simulink model "RotaryWingSim"  (Simulink 4.00)
settings: Solver=ode15s  StartTime=0.0  StopTime=simTime  RelTol=1e-10
values from neighbouring files (symbols this model uses):
  A1STrim = A1S    [AcFrcMmtSummationOutF.m]    (also in RotaryWingSimStart.m = AB1CP(1) + A1CL)
  B1STrim = B1S    [AcFrcMmtSummationOutF.m]    (also in RotaryWingSimStart.m = AB1CP(2) + B1CL)
  C5 = dthetomddelc    [RotaryWingSimStart.m]
  dla = u(2)    [D2ABcpSfunc.m]    (also in RotaryWingSimStart.m = trmOut(3))
  dlc = trmOut(1)    [RotaryWingSimStart.m]
  dlcTrim = dlc    [RotaryWingSimStart.m]
  dle = u(1)    [D2ABcpSfunc.m]    (also in HorizStabFrcMmtSFunc.m = u(7); RotaryWingSimStart.m = trmOut(2))
  dlp = u(7)    [FinFrcMmtSFunc.m]    (also in RotaryWingSimStart.m = trmOut(4); TailRotorFrcMmtSFunc.m)
  dlt = u(4)    [PropellerFrcMmtSFunc.m]    (also in RotaryWingSimStart.m = trmOut(5); acTrim3DFM.m = real(deltt(i)))
  fZMRTrim = -trmOut(9)    [RotaryWingSimStart.m]
  gamRot = 10    [LongitudinalStabilityBensen.m]    (also in N6NNeval.m = 12.5; RotaryWingSimStart.m = gamRot*rhoAir/rhoAirN)
  kB = K_l*tauB    [RotaryWingSimStart.m]
  oMTrim = trmOut(8)    [RotaryWingSimStart.m]
  phiTrim = trmOut(6)    [RotaryWingSimStart.m]
  psiTrim = aE(3)    [RotaryWingSimStart.m]
  tauAgLp = 1.0e-12    (= 1e-12)    [RotaryWingSimStart.m]
  thtaTrim = trmOut(7)    [RotaryWingSimStart.m]
  vE = [xh,0,0]    [RotaryWingSimStart.m]    (also in ac6DofFunc.m = vOut(2))
undefined symbols (not defined in the file or in its folder): A1CL, B1CL, d2ABCP, dlaStp, dlcStp, dleStp, dlpStp, dTstp, fStp1, PIDcllt, PIDphi, PIDpsi, PIDthta, tauB, tauC, tStp, uBStrt, vBStrt, wBStrt
libraries: simulink3 x1
settings Model: LastModifiedBy=jhumt  SaveState=on  InitialState=xFinal  SaveFinalState=on  RTWOptions="-aEnforceIntegerDowncast=1 -aExtMode=0 -aFoldNonRolledExpr=1 -aForceParamTrailComments=0 -aGenerateComments=1 -aIgnoreCustomStorageClasses=1 -aIncHierarchyInIds=0 -aInlineInvariantSignals=0 -aLocalBlockOutputs=1 -aLogVarNameModifier=\"rt_\" -aRTWVerbose=1 -aRollThreshold=5 -aShowEliminatedStatements=1"

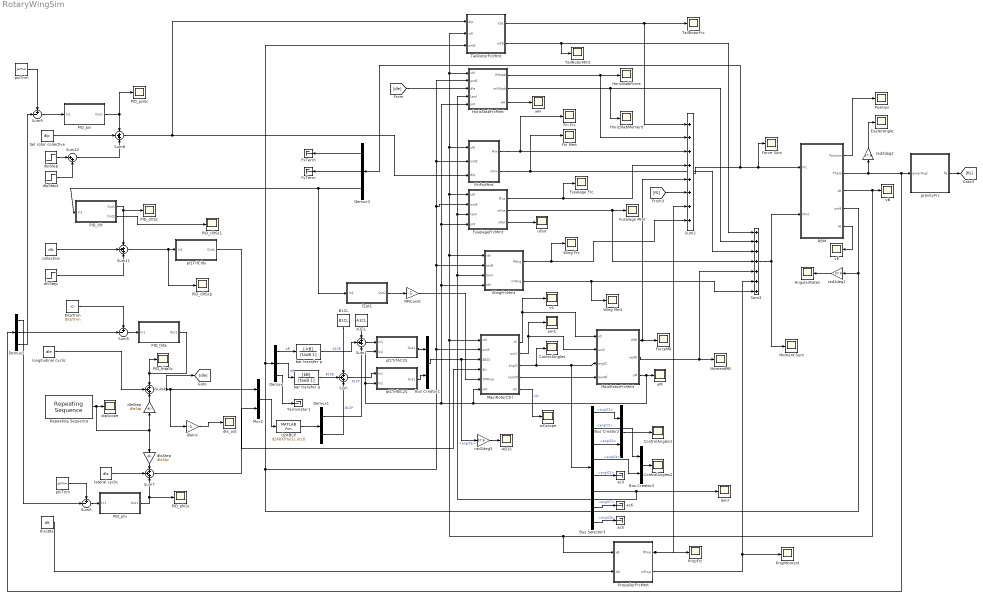
== system RotaryWingSim ==
  A1CL : Constant  Orientation=down  Value=A1CL
  AB1S : Scope
      settings: TimeRange=auto  YMin=-13  YMax=0  SaveToWorkspace=off  SaveName=ScopeData4  LimitDataPoints=on  MaxDataPoints=5000
  AngularRates : Scope
      settings: TimeRange=20  YMin=-12.5  YMax=15  SaveToWorkspace=off  SaveName=ScopeData20  LimitDataPoints=on  MaxDataPoints=25000
  B1CL : Constant  Orientation=down  Value=B1CL
  Bus Creator1 : BusCreator  Inputs=2
  Bus Creator2 : BusCreator  Inputs=2
  Bus Creator3 : BusCreator  Inputs=2
  Bus Selector3 : BusSelector  OutputSignals=anglC1,anglC2,anglC3,anglC4,anglC5,anglC6,anglC7,anglC8  MuxedOutput=off
  ControlAngles : Scope
      settings: TimeRange=auto  YMin=-0.035  YMax=0.065  SaveToWorkspace=off  LimitDataPoints=on  MaxDataPoints=5000
  ControlAngles1 : Scope
      settings: TimeRange=auto  YMin=0.043  YMax=0.064  SaveToWorkspace=off  SaveName=ScopeData33  LimitDataPoints=on  MaxDataPoints=5000
  ControlAngles2 : Scope
      settings: TimeRange=auto  YMin=-0.07  YMax=0.13  SaveToWorkspace=off  SaveName=ScopeData34  LimitDataPoints=on  MaxDataPoints=5000
  Demux : Demux  Outputs=3  BusSelectionMode=off
  Demux1 : Demux  Outputs=2  BusSelectionMode=off
  Demux2 : Demux  Outputs=3  BusSelectionMode=off
  Demux3 : Demux  Orientation=left  Outputs=3  BusSelectionMode=off
  EuelerAngle : Scope
      settings: TimeRange=auto  YMin=-7  YMax=7  SaveToWorkspace=off  SaveName=ScopeData17  LimitDataPoints=on  MaxDataPoints=25000
  Fin Frc : Scope
      settings: TimeRange=auto  YMin=-200  YMax=150  SaveToWorkspace=off  SaveName=ScopeData12  LimitDataPoints=on  MaxDataPoints=5000
  Fin Mmt : Scope
      settings: TimeRange=auto  YMin=-5  YMax=5  SaveToWorkspace=off  SaveName=ScopeData13  LimitDataPoints=on  MaxDataPoints=25000
  FinFrcMmt : Subsystem
      settings: RTWFcnNameOpts=Auto  RTWFileNameOpts=Auto
  Force Sum : Scope
      settings: TimeRange=0.02560000000000007  YMin=-0.0507109  YMax=0.0687204  SaveToWorkspace=off  SaveName=ScopeData15  LimitDataPoints=on  MaxDataPoints=5000
  ForceMR : Scope
      settings: TimeRange=30  YMin=-80000  YMax=5000  SaveToWorkspace=off  SaveName=ScopeData6  LimitDataPoints=on  MaxDataPoints=5000
  Fuselage Frc : Scope
      settings: TimeRange=auto  YMin=-5  YMax=5  SaveToWorkspace=off  SaveName=ScopeData10  LimitDataPoints=on  MaxDataPoints=5000
  Fuselage Mmt : Scope
      settings: TimeRange=auto  YMin=-175  YMax=25  SaveToWorkspace=off  SaveName=ScopeData11  LimitDataPoints=on  MaxDataPoints=5000
  FuselageFrcMmt : Subsystem
      settings: RTWFcnNameOpts=Auto  RTWFileNameOpts=Auto
  FxTerm : Terminator
  FyTerm : Terminator
  HorizStabForce : Scope
      settings: TimeRange=auto  YMin=-100  YMax=1200  SaveToWorkspace=off  SaveName=ScopeData18  LimitDataPoints=on  MaxDataPoints=5000
  HorizStabFrcMmt : Subsystem
      settings: RTWFcnNameOpts=Auto  RTWFileNameOpts=Auto
  HorizStabMoment : Scope
      settings: TimeRange=auto  YMin=0  YMax=450  SaveToWorkspace=off  SaveName=ScopeData19  LimitDataPoints=on  MaxDataPoints=25000
  MRConst : Gain  Gain=-1  Multiplication=Element-wise(K.*u)  SaturateOnIntegerOverflow=on
  MainRotorCtrl : Subsystem
      settings: RTWFcnNameOpts=Auto  RTWFileNameOpts=Auto
  MainRotorFrcMmt : Subsystem
      settings: RTWFcnNameOpts=Auto  RTWFileNameOpts=Auto
  Moment Sum : Scope
      settings: TimeRange=auto  YMin=-5  YMax=45  SaveToWorkspace=off  SaveName=ScopeData14  LimitDataPoints=on  MaxDataPoints=5000
  MomentMR : Scope
      settings: TimeRange=auto  YMin=-2250  YMax=500  SaveToWorkspace=off  SaveName=ScopeData5  LimitDataPoints=on  MaxDataPoints=25000
  Mux2 : Mux  Inputs=2
  PID_cllt : Subsystem
      settings: RTWFcnNameOpts=Auto  RTWFileNameOpts=Auto
  PID_clltSc : Scope
      settings: TimeRange=auto  YMin=-1  YMax=1  SaveToWorkspace=off  SaveName=ScopeData29  LimitDataPoints=on  MaxDataPoints=5000
  PID_clltSc1 : Scope
      settings: TimeRange=auto  YMin=-26  YMax=-15  SaveToWorkspace=off  SaveName=ScopeData30  LimitDataPoints=on  MaxDataPoints=5000
  PID_clltScp : Scope
      settings: TimeRange=auto  YMin=0.19401  YMax=0.19407  SaveToWorkspace=off  SaveName=ScopeData22  LimitDataPoints=on  MaxDataPoints=5000
  PID_phi : Subsystem
      settings: RTWFcnNameOpts=Auto  RTWFileNameOpts=Auto
  PID_phiSc : Scope
      settings: TimeRange=auto  YMin=-5  YMax=5  SaveToWorkspace=off  SaveName=ScopeData26  LimitDataPoints=on  MaxDataPoints=5000
  PID_psi : Subsystem
      settings: RTWFcnNameOpts=Auto  RTWFileNameOpts=Auto
  PID_psiSc : Scope
      settings: TimeRange=auto  YMin=-0.015  YMax=0.0025  SaveToWorkspace=off  SaveName=ScopeData25  LimitDataPoints=on  MaxDataPoints=5000
  PID_thta : Subsystem
      settings: RTWFcnNameOpts=Auto  RTWFileNameOpts=Auto
  PID_thtaSc : Scope
      settings: TimeRange=auto  YMin=-4.5  YMax=1  SaveToWorkspace=off  SaveName=ScopeData24  LimitDataPoints=on  MaxDataPoints=5000
  Position : Scope
      settings: TimeRange=auto  YMin=-500  YMax=1500  SaveToWorkspace=off  SaveName=ScopeData16  LimitDataPoints=on  MaxDataPoints=25000
  PropFrc : Scope
      settings: TimeRange=auto  YMin=0  YMax=350  SaveToWorkspace=off  SaveName=ScopeData36  LimitDataPoints=on  MaxDataPoints=5000
  PropMoment : Scope
      settings: TimeRange=auto  YMin=0  YMax=15  SaveToWorkspace=off  SaveName=ScopeData35  LimitDataPoints=on  MaxDataPoints=5000
  PropellerFrcMmt : Subsystem
      settings: RTWFcnNameOpts=Auto  RTWFileNameOpts=Auto
  RBM : Subsystem
      settings: RTWFcnNameOpts=Auto  RTWFileNameOpts=Auto
  Repeating Sequence : simulink3/Sources/Repeating Sequence  rep_seq_t=fStp1(1,:)  rep_seq_y=fStp1(2,:)
  Sum{,1,4,7..8,11} (6 alike) : Sum  Inputs=+++  SaturateOnIntegerOverflow=on
  Sum12 : Sum  Inputs=|++  SaturateOnIntegerOverflow=on
  Sum2 : Sum  Inputs=++++++++  SaturateOnIntegerOverflow=on
  Sum3 : Sum  Inputs=+++++++  SaturateOnIntegerOverflow=on
  Sum5 : Sum  Inputs=+-|  SaturateOnIntegerOverflow=on
  Sum6 : Sum  Inputs=+-|  SaturateOnIntegerOverflow=on
  Sum9 : Sum  Inputs=+-|  SaturateOnIntegerOverflow=on
  TailRotorFrc : Scope
      settings: TimeRange=auto  YMin=-5  YMax=5  SaveToWorkspace=off  SaveName=ScopeData8  LimitDataPoints=on  MaxDataPoints=5000
  TailRotorFrcMmt : Subsystem
      settings: RTWFcnNameOpts=Auto  RTWFileNameOpts=Auto
  TailRotorMmt : Scope
      settings: TimeRange=auto  YMin=-50000  YMax=200000  SaveToWorkspace=off  SaveName=ScopeData9  LimitDataPoints=on  MaxDataPoints=5000
  Terminator1 : Terminator
  Wing Frc : Scope
      settings: TimeRange=auto  YMin=-1750  YMax=0  SaveToWorkspace=off  SaveName=ScopeData39  LimitDataPoints=on  MaxDataPoints=5000
  Wing Mmt : Scope
      settings: TimeRange=auto  YMin=-7.5  YMax=15  SaveToWorkspace=off  SaveName=ScopeData38  LimitDataPoints=on  MaxDataPoints=5000
  WingFrcMmt : Subsystem
      settings: RTWFcnNameOpts=Auto  RTWFileNameOpts=Auto
  ac3 : Terminator
  ac5 : Terminator
  ac6 : Terminator
  bar transfer p : TransferFcn  Numerator=[-kB]  Denominator=[tauB 1]  AbsoluteTolerance=auto  Realization=auto
  bar transfer q : TransferFcn  Numerator=[kB]  Denominator=[tauB 1]  AbsoluteTolerance=auto  Realization=auto
  collective : Constant  Value=dlc
  d2ABCP : MATLABFcn  MATLABFcn=d2ABCP(u(1),u(2))  OutputDimensions=-1  OutputSignalType=auto  Output1D=on
  dlaStep : Gain  Orientation=down  Gain=dlaStp  Multiplication=Element-wise(K.*u)  SaturateOnIntegerOverflow=on
  dlcStep : Step  Time=tStp  Before=0  After=dlcStp  SampleTime=0
  dleInv : Gain  Gain=-1  Multiplication=Element-wise(K.*u)  SaturateOnIntegerOverflow=on
  dleStep : Gain  Orientation=up  Gain=dleStp  Multiplication=Element-wise(K.*u)  SaturateOnIntegerOverflow=on
  dle_out : Scope
      settings: TimeRange=auto  YMin=-125  YMax=75  SaveToWorkspace=off  SaveName=ScopeData32  LimitDataPoints=on  MaxDataPoints=15000
  dlpStep : Step  Time=tStp  Before=0  After=dlpStp  SampleTime=0
  dlpStep1 : Step  Time=tStp + dTstp  Before=0  After=- dlpStp  SampleTime=0
  fZpt1 : Subsystem
      settings: RTWFcnNameOpts=Auto  RTWFileNameOpts=Auto
  gravityFrc : Subsystem
      settings: RTWFcnNameOpts=Auto  RTWFileNameOpts=Auto
  lamI : Scope
      settings: TimeRange=auto  YMin=0  YMax=350  SaveToWorkspace=off  SaveName=ScopeData3  LimitDataPoints=on  MaxDataPoints=5000
  lateral cyclic : Constant  Value=dla
  longitudinal cyclic : Constant  Value=dle
  oM : Scope
      settings: TimeRange=auto  YMin=31  YMax=42  SaveToWorkspace=off  SaveName=ScopeData7  LimitDataPoints=on  MaxDataPoints=25000
  omC : Scope
      settings: TimeRange=auto  YMin=-5  YMax=5  SaveToWorkspace=off  SaveName=ScopeData2  LimitDataPoints=on  MaxDataPoints=5000
  phiTrim : Constant  Value=phiTrim
  psiTrim : Constant  Value=psiTrim
  pt1TrfAC2S : Subsystem
      settings: RTWFcnNameOpts=Auto  RTWFileNameOpts=Auto
  pt1TrfBC2S : Subsystem
      settings: RTWFcnNameOpts=Auto  RTWFileNameOpts=Auto
  pt1TrfClltv : Subsystem
      settings: RTWFcnNameOpts=Auto  RTWFileNameOpts=Auto
  rad2deg1 : Gain  Orientation=left  Gain=57.6  Multiplication=Element-wise(K.*u)  SaturateOnIntegerOverflow=on
  rad2deg2 : Gain  Orientation=up  Gain=57.6  Multiplication=Element-wise(K.*u)  SaturateOnIntegerOverflow=on
  rad2deg3 : Gain  Gain=57.6  Multiplication=Element-wise(K.*u)  SaturateOnIntegerOverflow=on
  stpScope : Scope
      settings: TimeRange=auto  YMin=-0.5  YMax=1.2  SaveToWorkspace=off  SaveName=ScopeData37  LimitDataPoints=on  MaxDataPoints=5000
  tail rotor collective : Constant  Value=dlp
  throttle : Constant  Value=dlt
  thtaTrim : Constant  Value=thtaTrim
  uOut : Scope
      settings: TimeRange=auto  YMin=-5  YMax=5  SaveToWorkspace=off  SaveName=ScopeData28  LimitDataPoints=on  MaxDataPoints=5000
  vB : Scope
      settings: TimeRange=auto  YMin=0  YMax=30  SaveToWorkspace=off  SaveName=ScopeData27  LimitDataPoints=on  MaxDataPoints=5000
  vC : Scope
      settings: TimeRange=auto  YMin=-5  YMax=5  SaveToWorkspace=off  SaveName=ScopeData  LimitDataPoints=on  MaxDataPoints=5000
  vE : Scope
      settings: TimeRange=auto  YMin=0  YMax=32.5  SaveToWorkspace=off  SaveName=ScopeData31  LimitDataPoints=on  MaxDataPoints=5000
  wCscope : Scope
      settings: TimeRange=auto  YMin=-5  YMax=5  SaveToWorkspace=off  SaveName=ScopeData21  LimitDataPoints=on  MaxDataPoints=5000
  wH : Scope
      settings: TimeRange=auto  YMin=-5  YMax=5  SaveToWorkspace=off  SaveName=ScopeData23  LimitDataPoints=on  MaxDataPoints=5000
  wires:
  Mux2/1 -> d2ABCP/1
  d2ABCP/1 -> Demux1/1
  Demux/1 -> bar transfer p/1  "pB"
  Demux/2 -> bar transfer q/1  "qB"
  bar transfer p/1 -> Sum1/2  "A1CB"
  bar transfer q/1 -> Sum/2  "B1CB"
  B1CL/1 -> Sum/1
  A1CL/1 -> Sum1/1
  Demux1/1 -> Sum1/3  "A1CP"
  Demux1/2 -> Sum/3  "B1CP"
  Sum1/1 -> pt1TrfAC2S/1(In1)
  Sum/1 -> pt1TrfBC2S/1(In1)
  pt1TrfBC2S/1(Out1) -> Bus Creator1/2
  pt1TrfAC2S/1(Out1) -> Bus Creator1/1
  MainRotorCtrl/4(lamNf) -> MainRotorFrcMmt/4(lamNf)
  pt1TrfClltv/1(Out1) -> MainRotorCtrl/4(dlc)
  Bus Creator1/1 -> MainRotorCtrl/3(AB1S), rad2deg3/1
  Demux/3 -> Terminator1/1
  MainRotorCtrl/1(vC) -> vC/1, MainRotorFrcMmt/1(vC)
  MainRotorCtrl/2(omC) -> omC/1, MainRotorFrcMmt/2(omC)
  MainRotorCtrl/3(anglC) -> ControlAngles/1, MainRotorFrcMmt/3(anglC), Bus Selector3/1
  MainRotorFrcMmt/2(mMR) -> Sum3/5, MomentMR/1
  MainRotorFrcMmt/1(fMR) -> ForceMR/1, Sum2/5
  tail rotor collective/1 -> Sum8/2
  TailRotorFrcMmt/2(mTR) -> Sum3/1, TailRotorMmt/1
  TailRotorFrcMmt/1(fTR) -> Sum2/1, TailRotorFrc/1
  FuselageFrcMmt/1(fFus) -> Sum2/4, Fuselage Frc/1
  FuselageFrcMmt/2(mFus) -> Sum3/4, Fuselage Mmt/1
  FinFrcMmt/1(fFin) -> Fin Frc/1, Sum2/3
  FinFrcMmt/2(mFin) -> Fin Mmt/1, Sum3/3
  [dle] -> HorizStabFrcMmt/3(dle)
  Sum2/1 -> Force Sum/1, RBM/1(Frc), Demux3/1
  HorizStabFrcMmt/1(fHStab) -> Sum2/2, HorizStabForce/1
  HorizStabFrcMmt/2(mHStab) -> Sum3/2, HorizStabMoment/1
  Sum3/1 -> Moment Sum/1, RBM/2(Mmt)
  RBM/2(Theta) -> gravityFrc/1(eulerAngl), Demux2/1, rad2deg2/1
  RBM/1(Position) -> Position/1
  [fG] -> Sum2/6
  gravityFrc/1(fG) -> [fG]
  HorizStabFrcMmt/3(wH) -> wH/1
  Sum4/1 -> [dle], Mux2/1, dleInv/1
  thtaTrim/1 -> Sum5/1
  Sum5/1 -> PID_thta/1(In1)
  Demux2/2 -> Sum5/2
  Demux2/1 -> Sum6/2
  Demux2/3 -> Sum9/2
  PID_thta/1(Out1) -> Sum4/1, PID_thtaSc/1
  phiTrim/1 -> Sum6/1
  Sum6/1 -> PID_phi/1(In1)
  Sum7/1 -> Mux2/2
  PID_phi/1(Out1) -> PID_phiSc/1, Sum7/3
  Sum8/1 -> TailRotorFrcMmt/1(dlp), FinFrcMmt/3(dlp)
  PID_psi/1(Out1) -> Sum8/1, PID_psiSc/1
  Sum9/1 -> PID_psi/1(In1)
  psiTrim/1 -> Sum9/1
  RBM/3(vB) -> vB/1, MainRotorCtrl/1(vW), FuselageFrcMmt/1(vW), FinFrcMmt/1(vW), HorizStabFrcMmt/1(vW), TailRotorFrcMmt/2(vW), WingFrcMmt/1(vW), PropellerFrcMmt/1(vB)
  FuselageFrcMmt/3(uOut) -> uOut/1
  collective/1 -> Sum11/2
  Sum11/1 -> pt1TrfClltv/1(In1), PID_clltScp/1
  PID_cllt/1(Out1) -> Sum11/1, PID_clltSc/1
  Demux3/1 -> FxTerm/1
  Demux3/2 -> FyTerm/1
  Demux3/3 -> PID_cllt/1(In1), fZpt1/1(In1)
  PID_cllt/2(Out2) -> PID_clltSc1/1
  RBM/5(vE) -> vE/1
  longitudinal cyclic/1 -> Sum4/2
  MainRotorCtrl/5(wC) -> wCscope/1  "vZc"
  RBM/4(omB) -> MainRotorCtrl/2(omB), FuselageFrcMmt/2(omB), FinFrcMmt/2(omB), HorizStabFrcMmt/2(omB), WingFrcMmt/2(omB), TailRotorFrcMmt/3(omB), Demux/1, rad2deg1/1
  rad2deg1/1 -> AngularRates/1
  dlcStep/1 -> Sum11/3
  dlpStep1/1 -> Sum12/2
  dlpStep/1 -> Sum12/1
  Sum12/1 -> Sum8/3
  lateral cyclic/1 -> Sum7/2
  dleStep/1 -> Sum4/3
  dlaStep/1 -> Sum7/1
  rad2deg2/1 -> EuelerAngle/1
  throttle/1 -> PropellerFrcMmt/2(dlt)
  PropellerFrcMmt/2(mProp) -> Sum3/6, PropMoment/1
  PropellerFrcMmt/1(fProp) -> Sum2/7, PropFrc/1
  MainRotorFrcMmt/3(oM) -> oM/1, pt1TrfAC2S/2(In2), pt1TrfBC2S/2(In2), WingFrcMmt/4(oM), FuselageFrcMmt/4(oM), HorizStabFrcMmt/5(oM), MainRotorCtrl/6(oM)
  Bus Selector3/5 -> ac3/1  "<anglC5>"
  Bus Selector3/7 -> ac6/1  "<anglC7>"
  Bus Selector3/8 -> ac5/1  "<anglC8>"
  Bus Creator2/1 -> ControlAngles1/1
  Bus Selector3/4 -> Bus Creator3/2  "<anglC4>"
  Bus Selector3/2 -> Bus Creator3/1  "<anglC2>"
  Bus Selector3/1 -> Bus Creator2/1  "<anglC1>"
  Bus Selector3/3 -> Bus Creator2/2  "<anglC3>"
  Bus Creator3/1 -> ControlAngles2/1
  rad2deg3/1 -> AB1S/1
  fZpt1/1(Out1) -> MRConst/1
  MRConst/1 -> MainRotorCtrl/5(TMRinp)
  WingFrcMmt/2(mWng) -> Sum3/7, Wing Mmt/1
  WingFrcMmt/1(fWng) -> Sum2/8, Wing Frc/1
  Repeating Sequence/1 -> stpScope/1, dleStep/1, dlaStep/1
  Bus Selector3/6 -> lamI/1, WingFrcMmt/3("lamI "), FuselageFrcMmt/3(lamI), HorizStabFrcMmt/4(lamI)  "<anglC6>"
  dleInv/1 -> dle_out/1

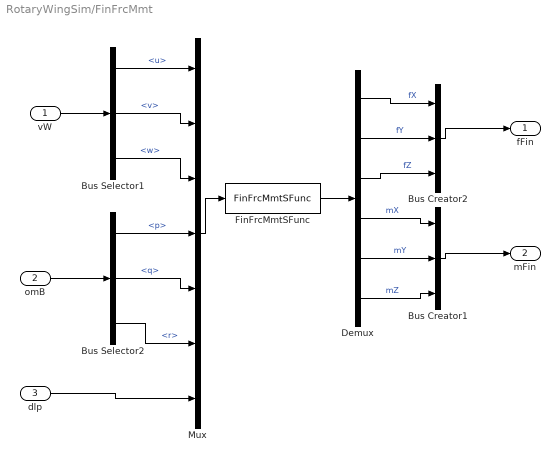
== system RotaryWingSim/FinFrcMmt ==
  vW : Inport  Port=1  LatchInput=off
  omB : Inport  Port=2  LatchInput=off
  dlp : Inport  Port=3  LatchInput=off
  Bus Creator1 : BusCreator  Inputs=3
  Bus Creator2 : BusCreator  Inputs=3
  Bus Selector1 : BusSelector  OutputSignals=u,v,w  MuxedOutput=off
  Bus Selector2 : BusSelector  OutputSignals=p,q,r  MuxedOutput=off
  Demux : Demux  Outputs=6  BusSelectionMode=off
  FinFrcMmtSFunc : S-Function  FunctionName=FinFrcMmtSFunc  PortCounts=[]  SFunctionModules=''
  Mux : Mux  Inputs=7
  fFin : Outport  Port=1
  mFin : Outport  Port=2
  wires:
  vW/1 -> Bus Selector1/1
  Bus Creator2/1 -> fFin/1
  FinFrcMmtSFunc/1 -> Demux/1
  Mux/1 -> FinFrcMmtSFunc/1
  Bus Selector1/2 -> Mux/2  "<v>"
  Bus Selector1/3 -> Mux/3  "<w>"
  omB/1 -> Bus Selector2/1
  Bus Selector2/1 -> Mux/4  "<p>"
  Bus Creator1/1 -> mFin/1
  Demux/1 -> Bus Creator2/1  "fX"
  Demux/2 -> Bus Creator2/2  "fY"
  Demux/3 -> Bus Creator2/3  "fZ"
  Demux/4 -> Bus Creator1/1  "mX"
  Demux/5 -> Bus Creator1/2  "mY"
  Demux/6 -> Bus Creator1/3  "mZ"
  Bus Selector2/2 -> Mux/5  "<q>"
  Bus Selector2/3 -> Mux/6  "<r>"
  Bus Selector1/1 -> Mux/1  "<u>"
  dlp/1 -> Mux/7

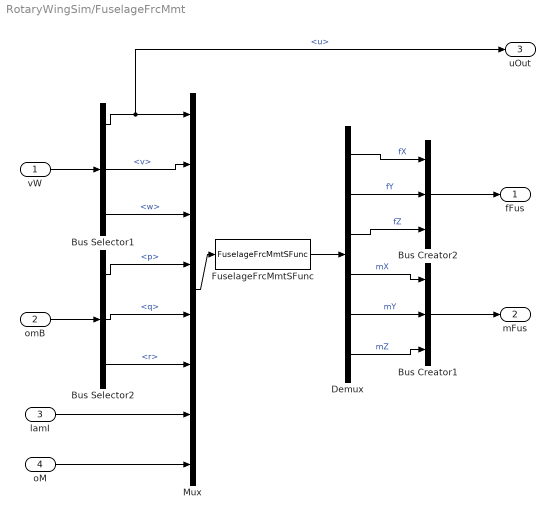
== system RotaryWingSim/FuselageFrcMmt ==
  vW : Inport  Port=1  LatchInput=off
  omB : Inport  Port=2  LatchInput=off
  lamI : Inport  Port=3  LatchInput=off
  oM : Inport  Port=4  LatchInput=off
  Bus Creator1 : BusCreator  Inputs=3
  Bus Creator2 : BusCreator  Inputs=3
  Bus Selector1 : BusSelector  OutputSignals=u,v,w  MuxedOutput=off
  Bus Selector2 : BusSelector  OutputSignals=p,q,r  MuxedOutput=off
  Demux : Demux  Outputs=6  BusSelectionMode=off
  FuselageFrcMmtSFunc : S-Function  FunctionName=FuselageFrcMmtSFunc  PortCounts=[]  SFunctionModules=''
  Mux : Mux  Inputs=8
  fFus : Outport  Port=1
  mFus : Outport  Port=2
  uOut : Outport  Port=3
  wires:
  vW/1 -> Bus Selector1/1
  Bus Creator2/1 -> fFus/1
  FuselageFrcMmtSFunc/1 -> Demux/1
  Mux/1 -> FuselageFrcMmtSFunc/1
  Bus Selector1/1 -> Mux/1, uOut/1  "<u>"
  Bus Selector1/2 -> Mux/2  "<v>"
  omB/1 -> Bus Selector2/1
  Bus Selector2/1 -> Mux/4  "<p>"
  Bus Selector2/2 -> Mux/5  "<q>"
  Bus Selector2/3 -> Mux/6  "<r>"
  Bus Creator1/1 -> mFus/1
  Demux/1 -> Bus Creator2/1  "fX"
  Demux/2 -> Bus Creator2/2  "fY"
  Demux/3 -> Bus Creator2/3  "fZ"
  Demux/4 -> Bus Creator1/1  "mX"
  Demux/5 -> Bus Creator1/2  "mY"
  Demux/6 -> Bus Creator1/3  "mZ"
  Bus Selector1/3 -> Mux/3  "<w>"
  lamI/1 -> Mux/7
  oM/1 -> Mux/8

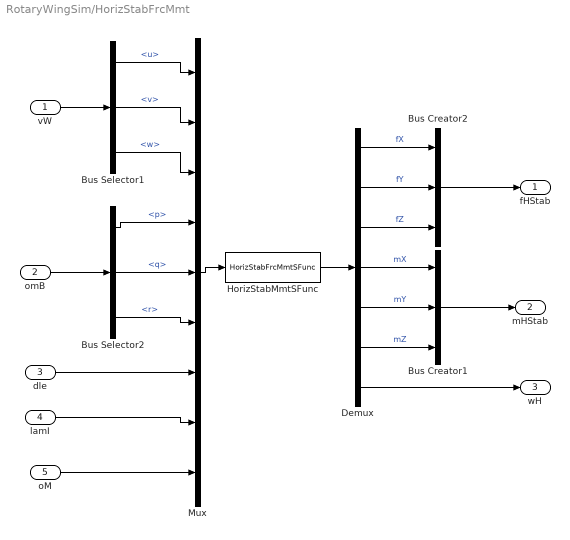
== system RotaryWingSim/HorizStabFrcMmt ==
  vW : Inport  Port=1  LatchInput=off
  omB : Inport  Port=2  LatchInput=off
  dle : Inport  Port=3  LatchInput=off
  lamI : Inport  Port=4  LatchInput=off
  oM : Inport  Port=5  LatchInput=off
  Bus Creator1 : BusCreator  Inputs=3
  Bus Creator2 : BusCreator  Inputs=3
  Bus Selector1 : BusSelector  OutputSignals=u,v,w  MuxedOutput=off
  Bus Selector2 : BusSelector  OutputSignals=p,q,r  MuxedOutput=off
  Demux : Demux  Outputs=7  BusSelectionMode=off
  HorizStabMmtSFunc : S-Function  FunctionName=HorizStabFrcMmtSFunc  PortCounts=[]  SFunctionModules=''
  Mux : Mux  Inputs=9
  fHStab : Outport  Port=1
  mHStab : Outport  Port=2
  wH : Outport  Port=3
  wires:
  vW/1 -> Bus Selector1/1
  Bus Creator2/1 -> fHStab/1
  HorizStabMmtSFunc/1 -> Demux/1
  Mux/1 -> HorizStabMmtSFunc/1
  Bus Selector1/1 -> Mux/1  "<u>"
  Bus Selector1/2 -> Mux/2  "<v>"
  Bus Selector1/3 -> Mux/3  "<w>"
  omB/1 -> Bus Selector2/1
  Bus Selector2/1 -> Mux/4  "<p>"
  Bus Selector2/2 -> Mux/5  "<q>"
  Bus Selector2/3 -> Mux/6  "<r>"
  Bus Creator1/1 -> mHStab/1
  Demux/1 -> Bus Creator2/1  "fX"
  Demux/2 -> Bus Creator2/2  "fY"
  Demux/3 -> Bus Creator2/3  "fZ"
  Demux/4 -> Bus Creator1/1  "mX"
  Demux/5 -> Bus Creator1/2  "mY"
  Demux/6 -> Bus Creator1/3  "mZ"
  dle/1 -> Mux/7
  lamI/1 -> Mux/8
  Demux/7 -> wH/1
  oM/1 -> Mux/9

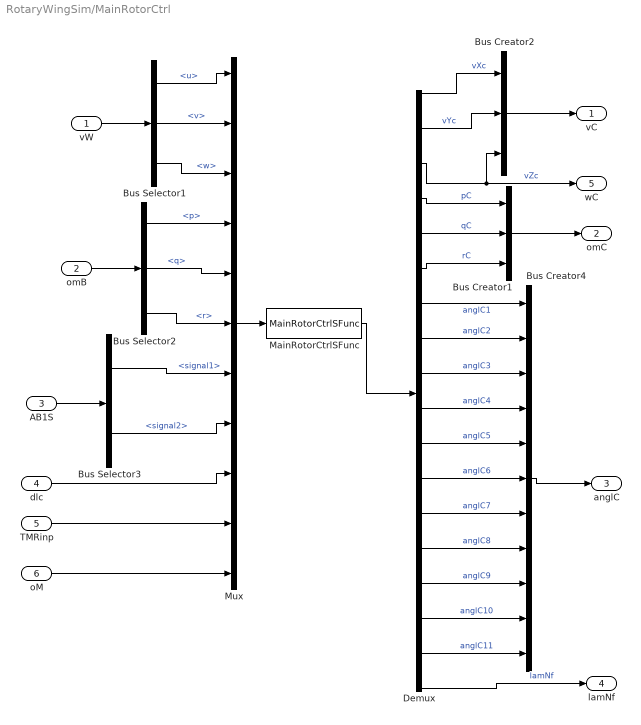
== system RotaryWingSim/MainRotorCtrl ==
  vW : Inport  Port=1  LatchInput=off
  omB : Inport  Port=2  LatchInput=off
  AB1S : Inport  Port=3  LatchInput=off
  dlc : Inport  Port=4  LatchInput=off
  TMRinp : Inport  Port=5  LatchInput=off
  oM : Inport  Port=6  LatchInput=off
  Bus Creator1 : BusCreator  Inputs=3
  Bus Creator2 : BusCreator  Inputs=3
  Bus Creator4 : BusCreator  Inputs=11
  Bus Selector1 : BusSelector  OutputSignals=u,v,w  MuxedOutput=off
  Bus Selector2 : BusSelector  OutputSignals=p,q,r  MuxedOutput=off
  Bus Selector3 : BusSelector  OutputSignals=signal1,signal2  MuxedOutput=off
  Demux : Demux  Outputs=18  BusSelectionMode=off
  MainRotorCtrlSFunc : S-Function  FunctionName=MainRotorCtrlSFunc  PortCounts=[]  SFunctionModules=''
  Mux : Mux  Inputs=11
  vC : Outport  Port=1
  omC : Outport  Port=2
  anglC : Outport  Port=3
  lamNf : Outport  Port=4
  wC : Outport  Port=5
  wires:
  vW/1 -> Bus Selector1/1
  Bus Creator2/1 -> vC/1
  dlc/1 -> Mux/9
  MainRotorCtrlSFunc/1 -> Demux/1
  Mux/1 -> MainRotorCtrlSFunc/1
  Bus Selector1/1 -> Mux/1  "<u>"
  Bus Selector1/2 -> Mux/2  "<v>"
  Bus Selector1/3 -> Mux/3  "<w>"
  omB/1 -> Bus Selector2/1
  Bus Selector2/1 -> Mux/4  "<p>"
  Bus Selector2/2 -> Mux/5  "<q>"
  Bus Selector2/3 -> Mux/6  "<r>"
  AB1S/1 -> Bus Selector3/1
  Bus Selector3/2 -> Mux/8  "<signal2>"
  Bus Selector3/1 -> Mux/7  "<signal1>"
  Bus Creator1/1 -> omC/1
  Demux/1 -> Bus Creator2/1  "vXc"
  Demux/2 -> Bus Creator2/2  "vYc"
  Demux/3 -> Bus Creator2/3, wC/1  "vZc"
  Demux/4 -> Bus Creator1/1  "pC"
  Demux/5 -> Bus Creator1/2  "qC"
  Demux/6 -> Bus Creator1/3  "rC"
  TMRinp/1 -> Mux/10
  oM/1 -> Mux/11
  Demux/7 -> Bus Creator4/1  "anglC1"
  Demux/8 -> Bus Creator4/2  "anglC2"
  Demux/9 -> Bus Creator4/3  "anglC3"
  Demux/10 -> Bus Creator4/4  "anglC4"
  Demux/11 -> Bus Creator4/5  "anglC5"
  Demux/12 -> Bus Creator4/6  "anglC6"
  Demux/13 -> Bus Creator4/7  "anglC7"
  Demux/14 -> Bus Creator4/8  "anglC8"
  Bus Creator4/1 -> anglC/1
  Demux/15 -> Bus Creator4/9  "anglC9"
  Demux/16 -> Bus Creator4/10  "anglC10"
  Demux/18 -> lamNf/1  "lamNf"
  Demux/17 -> Bus Creator4/11  "anglC11"

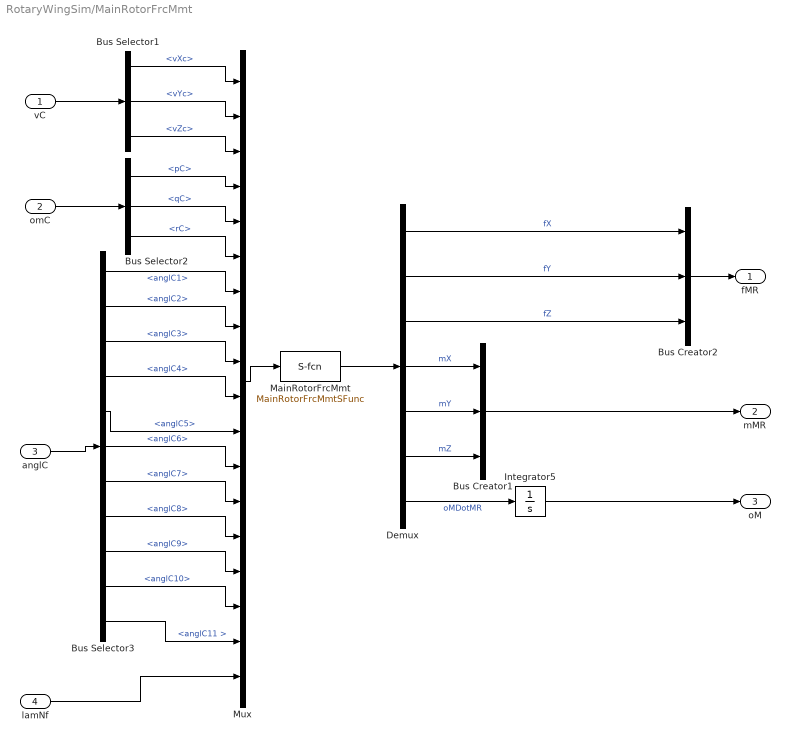
== system RotaryWingSim/MainRotorFrcMmt ==
  vC : Inport  Port=1  LatchInput=off
  omC : Inport  Port=2  LatchInput=off
  anglC : Inport  Port=3  LatchInput=off
  lamNf : Inport  Port=4  LatchInput=off
  Bus Creator1 : BusCreator  Inputs=3
  Bus Creator2 : BusCreator  Inputs=3
  Bus Selector1 : BusSelector  OutputSignals=vXc,vYc,vZc  MuxedOutput=off
  Bus Selector2 : BusSelector  OutputSignals=pC,qC,rC  MuxedOutput=off
  Bus Selector3 : BusSelector  OutputSignals=anglC1,anglC2,anglC3,anglC4,anglC5,anglC6,anglC7,anglC8,anglC9,anglC10,anglC11  MuxedOutput=off
  Demux : Demux  Outputs=7  BusSelectionMode=off
  Integrator5 : Integrator  ExternalReset=none  InitialConditionSource=internal  InitialCondition=oMTrim  LimitOutput=off  UpperSaturationLimit=inf  LowerSaturationLimit=-inf  ShowSaturationPort=off  ShowStatePort=off  AbsoluteTolerance=auto
  MainRotorFrcMmt : S-Function  FunctionName=MainRotorFrcMmtSFunc  PortCounts=[]  SFunctionModules=''
  Mux : Mux  Inputs=18
  fMR : Outport  Port=1
  mMR : Outport  Port=2
  oM : Outport  Port=3
  wires:
  vC/1 -> Bus Selector1/1
  omC/1 -> Bus Selector2/1
  anglC/1 -> Bus Selector3/1
  Bus Selector1/1 -> Mux/1  "<vXc>"
  Bus Selector1/2 -> Mux/2  "<vYc>"
  Bus Selector1/3 -> Mux/3  "<vZc>"
  Bus Selector2/1 -> Mux/4  "<pC>"
  Bus Selector2/2 -> Mux/5  "<qC>"
  Bus Selector2/3 -> Mux/6  "<rC>"
  Bus Selector3/2 -> Mux/8  "<anglC2>"
  Bus Selector3/3 -> Mux/9  "<anglC3>"
  Bus Selector3/1 -> Mux/7  "<anglC1>"
  Bus Selector3/4 -> Mux/10  "<anglC4>"
  Bus Selector3/5 -> Mux/11  "<anglC5>"
  Bus Creator2/1 -> fMR/1
  Bus Creator1/1 -> mMR/1
  Demux/1 -> Bus Creator2/1  "fX"
  Demux/2 -> Bus Creator2/2  "fY"
  Demux/4 -> Bus Creator1/1  "mX"
  Demux/5 -> Bus Creator1/2  "mY"
  Demux/6 -> Bus Creator1/3  "mZ"
  Mux/1 -> MainRotorFrcMmt/1
  MainRotorFrcMmt/1 -> Demux/1
  Demux/7 -> Integrator5/1  "oMDotMR"
  Integrator5/1 -> oM/1
  Bus Selector3/6 -> Mux/12  "<anglC6>"
  Bus Selector3/7 -> Mux/13  "<anglC7>"
  Bus Selector3/8 -> Mux/14  "<anglC8>"
  Bus Selector3/9 -> Mux/15  "<anglC9>"
  Bus Selector3/10 -> Mux/16  "<anglC10>"
  Demux/3 -> Bus Creator2/3  "fZ"
  lamNf/1 -> Mux/18
  Bus Selector3/11 -> Mux/17  "<anglC11 >"

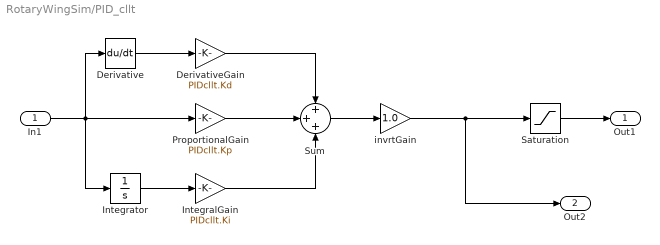
== system RotaryWingSim/PID_cllt ==
  In1 : Inport  Port=1  LatchInput=off
  Derivative : Derivative
  DerivativeGain : Gain  Gain=PIDcllt.Kd  Multiplication=Element-wise(K.*u)  SaturateOnIntegerOverflow=on
  IntegralGain : Gain  Gain=PIDcllt.Ki  Multiplication=Element-wise(K.*u)  SaturateOnIntegerOverflow=on
  Integrator : Integrator  ExternalReset=none  InitialConditionSource=internal  InitialCondition=0  LimitOutput=off  UpperSaturationLimit=inf  LowerSaturationLimit=-inf  ShowSaturationPort=off  ShowStatePort=off  AbsoluteTolerance=auto
  ProportionalGain : Gain  Gain=PIDcllt.Kp  Multiplication=Element-wise(K.*u)  SaturateOnIntegerOverflow=on
  Saturation : Saturate  UpperLimit=PIDcllt.zUpr  LowerLimit=PIDcllt.zLwr  LinearizeAsGain=on
  Sum : Sum  Inputs=+++  SaturateOnIntegerOverflow=on
  invrtGain : Gain  Gain=1.0  Multiplication=Element-wise(K.*u)  SaturateOnIntegerOverflow=on
  Out1 : Outport  Port=1
  Out2 : Outport  Port=2
  wires:
  Sum/1 -> invrtGain/1
  DerivativeGain/1 -> Sum/1
  IntegralGain/1 -> Sum/3
  Integrator/1 -> IntegralGain/1
  Derivative/1 -> DerivativeGain/1
  Saturation/1 -> Out1/1
  In1/1 -> Integrator/1, Derivative/1, ProportionalGain/1
  invrtGain/1 -> Saturation/1, Out2/1
  ProportionalGain/1 -> Sum/2

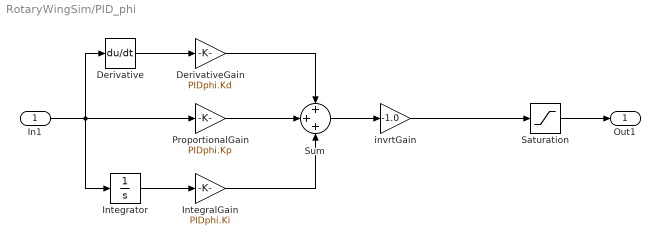
== system RotaryWingSim/PID_phi ==
  In1 : Inport  Port=1  LatchInput=off
  Derivative : Derivative
  DerivativeGain : Gain  Gain=PIDphi.Kd  Multiplication=Element-wise(K.*u)  SaturateOnIntegerOverflow=on
  IntegralGain : Gain  Gain=PIDphi.Ki  Multiplication=Element-wise(K.*u)  SaturateOnIntegerOverflow=on
  Integrator : Integrator  ExternalReset=none  InitialConditionSource=internal  InitialCondition=0  LimitOutput=off  UpperSaturationLimit=inf  LowerSaturationLimit=-inf  ShowSaturationPort=off  ShowStatePort=off  AbsoluteTolerance=auto
  ProportionalGain : Gain  Gain=PIDphi.Kp  Multiplication=Element-wise(K.*u)  SaturateOnIntegerOverflow=on
  Saturation : Saturate  UpperLimit=PIDphi.dlaUpr  LowerLimit=PIDphi.dlaLwr  LinearizeAsGain=on
  Sum : Sum  Inputs=+++  SaturateOnIntegerOverflow=on
  invrtGain : Gain  Gain=-1.0  Multiplication=Element-wise(K.*u)  SaturateOnIntegerOverflow=on
  Out1 : Outport  Port=1
  wires:
  Sum/1 -> invrtGain/1
  DerivativeGain/1 -> Sum/1
  IntegralGain/1 -> Sum/3
  ProportionalGain/1 -> Sum/2
  Integrator/1 -> IntegralGain/1
  Derivative/1 -> DerivativeGain/1
  Saturation/1 -> Out1/1
  In1/1 -> Integrator/1, Derivative/1, ProportionalGain/1
  invrtGain/1 -> Saturation/1

== system RotaryWingSim/PID_psi ==
  In1 : Inport  Port=1  LatchInput=off
  Derivative : Derivative
  DerivativeGain : Gain  Gain=PIDpsi.Kd  Multiplication=Element-wise(K.*u)  SaturateOnIntegerOverflow=on
  IntegralGain : Gain  Gain=PIDpsi.Ki  Multiplication=Element-wise(K.*u)  SaturateOnIntegerOverflow=on
  Integrator : Integrator  ExternalReset=none  InitialConditionSource=internal  InitialCondition=0  LimitOutput=off  UpperSaturationLimit=inf  LowerSaturationLimit=-inf  ShowSaturationPort=off  ShowStatePort=off  AbsoluteTolerance=auto
  ProportionalGain : Gain  Gain=PIDpsi.Kp  Multiplication=Element-wise(K.*u)  SaturateOnIntegerOverflow=on
  Saturation : Saturate  UpperLimit=PIDpsi.dlpUpr  LowerLimit=PIDpsi.dlpLwr  LinearizeAsGain=on
  Sum : Sum  Inputs=+++  SaturateOnIntegerOverflow=on
  invrtGain : Gain  Gain=-1.0  Multiplication=Element-wise(K.*u)  SaturateOnIntegerOverflow=on
  Out1 : Outport  Port=1
  wires:
  Sum/1 -> invrtGain/1
  DerivativeGain/1 -> Sum/1
  IntegralGain/1 -> Sum/3
  ProportionalGain/1 -> Sum/2
  Integrator/1 -> IntegralGain/1
  Derivative/1 -> DerivativeGain/1
  Saturation/1 -> Out1/1
  In1/1 -> Integrator/1, Derivative/1, ProportionalGain/1
  invrtGain/1 -> Saturation/1

== system RotaryWingSim/PID_thta ==
  In1 : Inport  Port=1  LatchInput=off
  Derivative : Derivative
  DerivativeGain : Gain  Gain=PIDthta.Kd  Multiplication=Element-wise(K.*u)  SaturateOnIntegerOverflow=on
  IntegralGain : Gain  Gain=PIDthta.Ki  Multiplication=Element-wise(K.*u)  SaturateOnIntegerOverflow=on
  Integrator : Integrator  ExternalReset=none  InitialConditionSource=internal  InitialCondition=0  LimitOutput=off  UpperSaturationLimit=inf  LowerSaturationLimit=-inf  ShowSaturationPort=off  ShowStatePort=off  AbsoluteTolerance=auto
  ProportionalGain : Gain  Gain=PIDthta.Kp  Multiplication=Element-wise(K.*u)  SaturateOnIntegerOverflow=on
  Saturation : Saturate  UpperLimit=PIDthta.dleUpr  LowerLimit=PIDthta.dleLwr  LinearizeAsGain=on
  Sum : Sum  Inputs=+++  SaturateOnIntegerOverflow=on
  invrtGain : Gain  Gain=-1.0  Multiplication=Element-wise(K.*u)  SaturateOnIntegerOverflow=on
  Out1 : Outport  Port=1
  wires:
  Sum/1 -> invrtGain/1
  DerivativeGain/1 -> Sum/1
  IntegralGain/1 -> Sum/3
  ProportionalGain/1 -> Sum/2
  Integrator/1 -> IntegralGain/1
  Derivative/1 -> DerivativeGain/1
  Saturation/1 -> Out1/1
  In1/1 -> Integrator/1, Derivative/1, ProportionalGain/1
  invrtGain/1 -> Saturation/1

== system RotaryWingSim/PropellerFrcMmt ==
  vB : Inport  Port=1  LatchInput=off
  dlt : Inport  Port=2  LatchInput=off
  Bus Creator1 : BusCreator  Inputs=3
  Bus Creator2 : BusCreator  Inputs=3
  Bus Selector1 : BusSelector  OutputSignals=u,v,w  MuxedOutput=off
  Demux : Demux  Outputs=6  BusSelectionMode=off
  Mux : Mux  Inputs=4
  PropellerFrcMmtSFunc : S-Function  FunctionName=PropellerFrcMmtSFunc  PortCounts=[]  SFunctionModules=''
  fProp : Outport  Port=1
  mProp : Outport  Port=2
  wires:
  vB/1 -> Bus Selector1/1
  Bus Creator2/1 -> fProp/1
  PropellerFrcMmtSFunc/1 -> Demux/1
  Mux/1 -> PropellerFrcMmtSFunc/1
  Bus Selector1/1 -> Mux/1  "<u>"
  Bus Selector1/2 -> Mux/2  "<v>"
  Bus Selector1/3 -> Mux/3  "<w>"
  Bus Creator1/1 -> mProp/1
  Demux/1 -> Bus Creator2/1  "fX"
  Demux/2 -> Bus Creator2/2  "fY"
  Demux/3 -> Bus Creator2/3  "fZ"
  Demux/4 -> Bus Creator1/1  "mX"
  Demux/5 -> Bus Creator1/2  "mY"
  Demux/6 -> Bus Creator1/3  "mZ"
  dlt/1 -> Mux/4

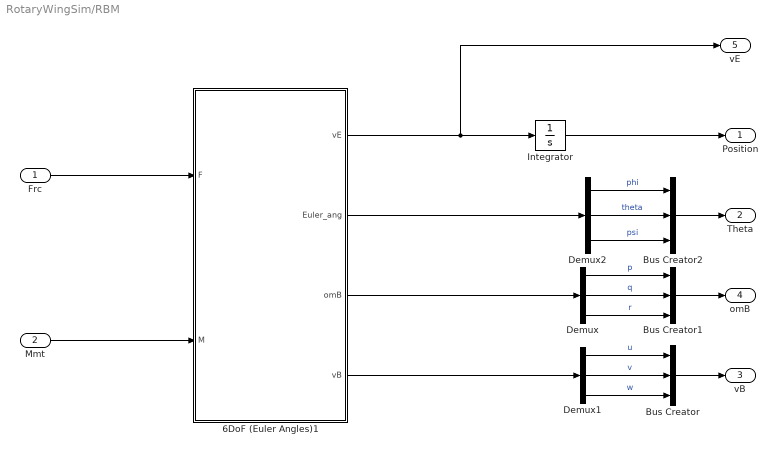
== system RotaryWingSim/RBM ==
  Frc : Inport  Port=1  LatchInput=off
  Mmt : Inport  Port=2  LatchInput=off
  6DoF (Euler Angles)1 : Subsystem
      settings: RTWFcnNameOpts=Auto  RTWFileNameOpts=Auto
  Bus Creator : BusCreator  Inputs=3
      settings: DisplayOption=none
  Bus Creator1 : BusCreator  Inputs=3
      settings: DisplayOption=none
  Bus Creator2 : BusCreator  Inputs=3
      settings: DisplayOption=none
  Demux : Demux  Outputs=3  BusSelectionMode=off
  Demux1 : Demux  Outputs=3  BusSelectionMode=off
  Demux2 : Demux  Outputs=3  BusSelectionMode=off
  Integrator : Integrator  ExternalReset=none  InitialConditionSource=internal  InitialCondition=0  LimitOutput=off  UpperSaturationLimit=inf  LowerSaturationLimit=-inf  ShowSaturationPort=off  ShowStatePort=off  AbsoluteTolerance=auto
  Position : Outport  Port=1
  Theta : Outport  Port=2
  vB : Outport  Port=3
  omB : Outport  Port=4
  vE : Outport  Port=5
  wires:
  Bus Creator/1 -> vB/1
  Bus Creator1/1 -> omB/1
  Demux1/1 -> Bus Creator/1  "u"
  Demux1/2 -> Bus Creator/2  "v"
  Demux1/3 -> Bus Creator/3  "w"
  Demux/1 -> Bus Creator1/1  "p"
  Demux/2 -> Bus Creator1/2  "q"
  Demux/3 -> Bus Creator1/3  "r"
  Bus Creator2/1 -> Theta/1
  6DoF (Euler Angles)1/3(omB) -> Demux/1
  6DoF (Euler Angles)1/4(vB) -> Demux1/1
  Integrator/1 -> Position/1
  6DoF (Euler Angles)1/2(Euler_ang) -> Demux2/1
  Demux2/1 -> Bus Creator2/1  "phi"
  Frc/1 -> 6DoF (Euler Angles)1/1(F)
  Mmt/1 -> 6DoF (Euler Angles)1/2(M)
  6DoF (Euler Angles)1/1(vE) -> Integrator/1, vE/1
  Demux2/2 -> Bus Creator2/2  "theta"
  Demux2/3 -> Bus Creator2/3  "psi"

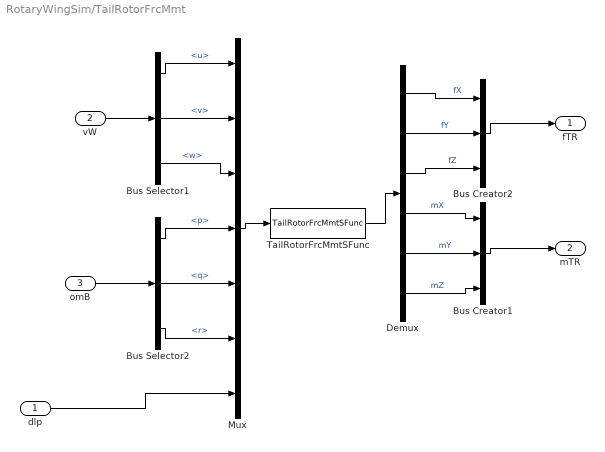
== system RotaryWingSim/TailRotorFrcMmt ==
  dlp : Inport  Port=1  LatchInput=off
  vW : Inport  Port=2  LatchInput=off
  omB : Inport  Port=3  LatchInput=off
  Bus Creator1 : BusCreator  Inputs=3
  Bus Creator2 : BusCreator  Inputs=3
  Bus Selector1 : BusSelector  OutputSignals=u,v,w  MuxedOutput=off
  Bus Selector2 : BusSelector  OutputSignals=p,q,r  MuxedOutput=off
  Demux : Demux  Outputs=6  BusSelectionMode=off
  Mux : Mux  Inputs=7
  TailRotorFrcMmtSFunc : S-Function  FunctionName=TailRotorFrcMmtSFunc  PortCounts=[]  SFunctionModules=''
  fTR : Outport  Port=1
  mTR : Outport  Port=2
  wires:
  vW/1 -> Bus Selector1/1
  Bus Creator2/1 -> fTR/1
  dlp/1 -> Mux/7
  TailRotorFrcMmtSFunc/1 -> Demux/1
  Mux/1 -> TailRotorFrcMmtSFunc/1
  Bus Selector1/1 -> Mux/1  "<u>"
  Bus Selector1/2 -> Mux/2  "<v>"
  Bus Selector1/3 -> Mux/3  "<w>"
  omB/1 -> Bus Selector2/1
  Bus Selector2/1 -> Mux/4  "<p>"
  Bus Selector2/2 -> Mux/5  "<q>"
  Bus Selector2/3 -> Mux/6  "<r>"
  Bus Creator1/1 -> mTR/1
  Demux/1 -> Bus Creator2/1  "fX"
  Demux/2 -> Bus Creator2/2  "fY"
  Demux/3 -> Bus Creator2/3  "fZ"
  Demux/4 -> Bus Creator1/1  "mX"
  Demux/5 -> Bus Creator1/2  "mY"
  Demux/6 -> Bus Creator1/3  "mZ"

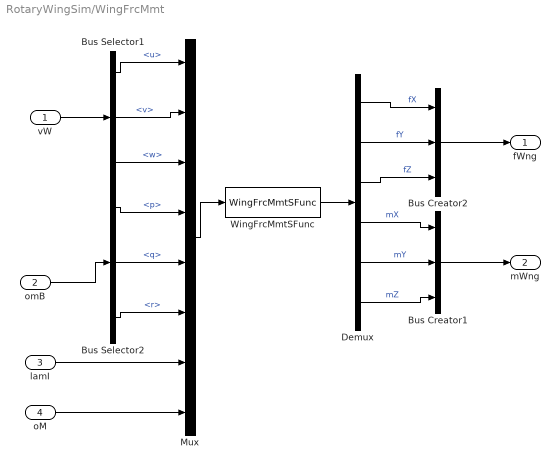
== system RotaryWingSim/WingFrcMmt ==
  vW : Inport  Port=1  LatchInput=off
  omB : Inport  Port=2  LatchInput=off
  "lamI " : Inport  Port=3  LatchInput=off
  oM : Inport  Port=4  LatchInput=off
  Bus Creator1 : BusCreator  Inputs=3
  Bus Creator2 : BusCreator  Inputs=3
  Bus Selector1 : BusSelector  OutputSignals=u,v,w  MuxedOutput=off
  Bus Selector2 : BusSelector  OutputSignals=p,q,r  MuxedOutput=off
  Demux : Demux  Outputs=6  BusSelectionMode=off
  Mux : Mux  Inputs=8
  WingFrcMmtSFunc : S-Function  FunctionName=WingFrcMmtSFunc  PortCounts=[]  SFunctionModules=''
  fWng : Outport  Port=1
  mWng : Outport  Port=2
  wires:
  vW/1 -> Bus Selector1/1
  Bus Creator2/1 -> fWng/1
  WingFrcMmtSFunc/1 -> Demux/1
  Mux/1 -> WingFrcMmtSFunc/1
  Bus Selector1/1 -> Mux/1  "<u>"
  Bus Selector1/2 -> Mux/2  "<v>"
  omB/1 -> Bus Selector2/1
  Bus Selector2/1 -> Mux/4  "<p>"
  Bus Selector2/2 -> Mux/5  "<q>"
  Bus Selector2/3 -> Mux/6  "<r>"
  Bus Creator1/1 -> mWng/1
  Demux/1 -> Bus Creator2/1  "fX"
  Demux/2 -> Bus Creator2/2  "fY"
  Demux/3 -> Bus Creator2/3  "fZ"
  Demux/4 -> Bus Creator1/1  "mX"
  Demux/5 -> Bus Creator1/2  "mY"
  Demux/6 -> Bus Creator1/3  "mZ"
  Bus Selector1/3 -> Mux/3  "<w>"
  "lamI "/1 -> Mux/7
  oM/1 -> Mux/8

== system RotaryWingSim/fZpt1 ==
  In1 : Inport  Port=1  LatchInput=off
  Integrator : Integrator  ExternalReset=none  InitialConditionSource=internal  InitialCondition=fZMRTrim  LimitOutput=off  UpperSaturationLimit=inf  LowerSaturationLimit=-inf  ShowSaturationPort=off  ShowStatePort=off  AbsoluteTolerance=auto
  Sum : Sum  Inputs=|+-  SaturateOnIntegerOverflow=on
  pt1Const : Gain  Gain=1  Multiplication=Element-wise(K.*u)  SaturateOnIntegerOverflow=on
  pt1Time : Gain  Gain=1/1.0e-10  Multiplication=Element-wise(K.*u)  SaturateOnIntegerOverflow=on
  Out1 : Outport  Port=1
  wires:
  In1/1 -> pt1Const/1
  Integrator/1 -> Sum/2, Out1/1
  pt1Const/1 -> Sum/1
  Sum/1 -> pt1Time/1
  pt1Time/1 -> Integrator/1

== system RotaryWingSim/gravityFrc ==
  eulerAngl : Inport  Port=1  LatchInput=off
  Bus Creator2 : BusCreator  Inputs=3
  Bus Selector1 : BusSelector  OutputSignals=phi,theta,psi  MuxedOutput=off
  Demux : Demux  Outputs=3  BusSelectionMode=off
  Mux : Mux  Inputs=3
  frcGSFunc : S-Function  FunctionName=frcGSFunc  PortCounts=[]  SFunctionModules=''
  fG : Outport  Port=1
  wires:
  eulerAngl/1 -> Bus Selector1/1
  Bus Creator2/1 -> fG/1
  frcGSFunc/1 -> Demux/1
  Mux/1 -> frcGSFunc/1
  Bus Selector1/1 -> Mux/1  "<phi>"
  Bus Selector1/2 -> Mux/2  "<theta>"
  Bus Selector1/3 -> Mux/3  "<psi >"
  Demux/1 -> Bus Creator2/1  "fX"
  Demux/2 -> Bus Creator2/2  "fY"
  Demux/3 -> Bus Creator2/3  "fZ"

== system RotaryWingSim/pt1TrfAC2S ==
  In1 : Inport  Port=1  LatchInput=off
  In2 : Inport  Port=2  LatchInput=off
  Gain : Gain  Gain=gamRot/16  Multiplication=Element-wise(K.*u)  SaturateOnIntegerOverflow=on
  Integrator : Integrator  ExternalReset=none  InitialConditionSource=internal  InitialCondition=A1STrim  LimitOutput=off  UpperSaturationLimit=inf  LowerSaturationLimit=-inf  ShowSaturationPort=off  ShowStatePort=off  AbsoluteTolerance=auto
  Product : Product  Inputs=/*  Multiplication=Element-wise(.*)  SaturateOnIntegerOverflow=on
  Sum : Sum  Inputs=|+-  SaturateOnIntegerOverflow=on
  Out1 : Outport  Port=1
  wires:
  Integrator/1 -> Sum/2, Out1/1
  In1/1 -> Sum/1
  Sum/1 -> Product/2
  Product/1 -> Integrator/1
  In2/1 -> Gain/1
  Gain/1 -> Product/1

== system RotaryWingSim/pt1TrfBC2S ==
  In1 : Inport  Port=1  LatchInput=off
  In2 : Inport  Port=2  LatchInput=off
  Gain : Gain  Gain=gamRot/16  Multiplication=Element-wise(K.*u)  SaturateOnIntegerOverflow=on
  Integrator : Integrator  ExternalReset=none  InitialConditionSource=internal  InitialCondition=B1STrim  LimitOutput=off  UpperSaturationLimit=inf  LowerSaturationLimit=-inf  ShowSaturationPort=off  ShowStatePort=off  AbsoluteTolerance=auto
  Product : Product  Inputs=/*  Multiplication=Element-wise(.*)  SaturateOnIntegerOverflow=on
  Sum : Sum  Inputs=|+-  SaturateOnIntegerOverflow=on
  Out1 : Outport  Port=1
  wires:
  Integrator/1 -> Sum/2, Out1/1
  In1/1 -> Sum/1
  Gain/1 -> Product/1
  In2/1 -> Gain/1
  Sum/1 -> Product/2
  Product/1 -> Integrator/1

== system RotaryWingSim/pt1TrfClltv ==
  In1 : Inport  Port=1  LatchInput=off
  Integrator : Integrator  ExternalReset=none  InitialConditionSource=internal  InitialCondition=dlcTrim*C5  LimitOutput=off  UpperSaturationLimit=inf  LowerSaturationLimit=-inf  ShowSaturationPort=off  ShowStatePort=off  AbsoluteTolerance=auto
  Sum : Sum  Inputs=|+-  SaturateOnIntegerOverflow=on
  pt1Const : Gain  Gain=C5  Multiplication=Element-wise(K.*u)  SaturateOnIntegerOverflow=on
  pt1Time : Gain  Gain=1/tauC  Multiplication=Element-wise(K.*u)  SaturateOnIntegerOverflow=on
  Out1 : Outport  Port=1
  wires:
  In1/1 -> pt1Const/1
  Integrator/1 -> Sum/2, Out1/1
  pt1Const/1 -> Sum/1
  Sum/1 -> pt1Time/1
  pt1Time/1 -> Integrator/1

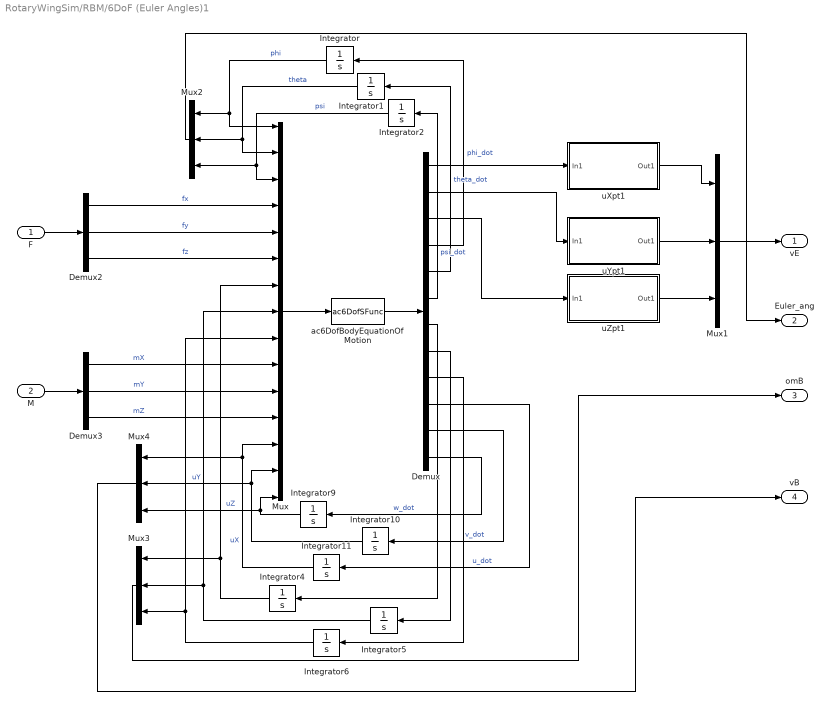
== system RotaryWingSim/RBM/6DoF (Euler Angles)1 ==
  F : Inport  Port=1  LatchInput=off
  M : Inport  Port=2  LatchInput=off
  Demux : Demux  Outputs=12  BusSelectionMode=off
  Demux2 : Demux  Outputs=3  BusSelectionMode=off
  Demux3 : Demux  Outputs=3  BusSelectionMode=off
  Integrator : Integrator  Orientation=left  ExternalReset=none  InitialConditionSource=internal  InitialCondition=phiTrim  LimitOutput=off  UpperSaturationLimit=inf  LowerSaturationLimit=-inf  ShowSaturationPort=off  ShowStatePort=off  AbsoluteTolerance=auto
  Integrator1 : Integrator  Orientation=left  ExternalReset=none  InitialConditionSource=internal  InitialCondition=thtaTrim  LimitOutput=off  UpperSaturationLimit=inf  LowerSaturationLimit=-inf  ShowSaturationPort=off  ShowStatePort=off  AbsoluteTolerance=auto
  Integrator10 : Integrator  Orientation=left  ExternalReset=none  InitialConditionSource=internal  InitialCondition=vBStrt  LimitOutput=off  UpperSaturationLimit=inf  LowerSaturationLimit=-inf  ShowSaturationPort=off  ShowStatePort=off  AbsoluteTolerance=auto
  Integrator11 : Integrator  Orientation=left  ExternalReset=none  InitialConditionSource=internal  InitialCondition=uBStrt  LimitOutput=off  UpperSaturationLimit=inf  LowerSaturationLimit=-inf  ShowSaturationPort=off  ShowStatePort=off  AbsoluteTolerance=auto
  Integrator2 : Integrator  Orientation=left  ExternalReset=none  InitialConditionSource=internal  InitialCondition=psiTrim  LimitOutput=off  UpperSaturationLimit=inf  LowerSaturationLimit=-inf  ShowSaturationPort=off  ShowStatePort=off  AbsoluteTolerance=auto
  Integrator4 : Integrator  Orientation=left  ExternalReset=none  InitialConditionSource=internal  InitialCondition=0  LimitOutput=off  UpperSaturationLimit=inf  LowerSaturationLimit=-inf  ShowSaturationPort=off  ShowStatePort=off  AbsoluteTolerance=auto
  Integrator5 : Integrator  Orientation=left  ExternalReset=none  InitialConditionSource=internal  InitialCondition=0  LimitOutput=off  UpperSaturationLimit=inf  LowerSaturationLimit=-inf  ShowSaturationPort=off  ShowStatePort=off  AbsoluteTolerance=auto
  Integrator6 : Integrator  Orientation=left  ExternalReset=none  InitialConditionSource=internal  InitialCondition=0  LimitOutput=off  UpperSaturationLimit=inf  LowerSaturationLimit=-inf  ShowSaturationPort=off  ShowStatePort=off  AbsoluteTolerance=auto
  Integrator9 : Integrator  Orientation=left  ExternalReset=none  InitialConditionSource=internal  InitialCondition=wBStrt  LimitOutput=off  UpperSaturationLimit=inf  LowerSaturationLimit=-inf  ShowSaturationPort=off  ShowStatePort=off  AbsoluteTolerance=auto
  Mux : Mux  Inputs=15
      settings: DisplayOption=none
  Mux1 : Mux  Inputs=3
      settings: DisplayOption=none
  Mux2 : Mux  Orientation=left  Inputs=3
      settings: DisplayOption=none
  Mux3 : Mux  Orientation=left  Inputs=3
      settings: DisplayOption=none
  Mux4 : Mux  Orientation=left  Inputs=3
      settings: DisplayOption=none
  ac6DofBodyEquationOfMotion : S-Function  FunctionName=ac6DofSFunc  PortCounts=[]  SFunctionModules=''
  uXpt1 : Subsystem
      settings: RTWFcnNameOpts=Auto  RTWFileNameOpts=Auto
  uYpt1 : Subsystem
      settings: RTWFcnNameOpts=Auto  RTWFileNameOpts=Auto
  uZpt1 : Subsystem
      settings: RTWFcnNameOpts=Auto  RTWFileNameOpts=Auto
  vE : Outport  Port=1
  Euler_ang : Outport  Port=2
  omB : Outport  Port=3
  vB : Outport  Port=4
  wires:
  ac6DofBodyEquationOfMotion/1 -> Demux/1
  Mux/1 -> ac6DofBodyEquationOfMotion/1
  Integrator4/1 -> Mux/7, Mux3/1
  Integrator/1 -> Mux/1, Mux2/1  "phi"
  Demux/2 -> uYpt1/1(In1)
  Demux/3 -> uZpt1/1(In1)
  Demux/4 -> Integrator/1  "phi_dot"
  Demux/5 -> Integrator1/1  "theta_dot"
  Demux/6 -> Integrator2/1  "psi_dot"
  Demux/7 -> Integrator4/1
  Demux/8 -> Integrator5/1
  Demux/9 -> Integrator6/1
  Integrator1/1 -> Mux/2, Mux2/2  "theta"
  Integrator2/1 -> Mux/3, Mux2/3  "psi"
  Integrator5/1 -> Mux/8, Mux3/2
  Integrator6/1 -> Mux/9, Mux3/3
  Demux3/1 -> Mux/10  "mX"
  Demux3/2 -> Mux/11  "mY"
  Demux3/3 -> Mux/12  "mZ"
  F/1 -> Demux2/1
  M/1 -> Demux3/1
  Mux1/1 -> vE/1
  Mux2/1 -> Euler_ang/1
  Mux3/1 -> omB/1
  Demux/10 -> Integrator11/1  "u_dot"
  Demux/11 -> Integrator10/1  "v_dot"
  Demux/12 -> Integrator9/1  "w_dot"
  Demux/1 -> uXpt1/1(In1)
  Demux2/1 -> Mux/4  "fx"
  Demux2/2 -> Mux/5  "fy"
  Demux2/3 -> Mux/6  "fz"
  Integrator9/1 -> Mux/15, Mux4/3  "uZ"
  Integrator10/1 -> Mux/14, Mux4/2  "uY"
  Integrator11/1 -> Mux/13, Mux4/1  "uX"
  Mux4/1 -> vB/1
  uZpt1/1(Out1) -> Mux1/3
  uYpt1/1(Out1) -> Mux1/2
  uXpt1/1(Out1) -> Mux1/1

== system RotaryWingSim/RBM/6DoF (Euler Angles)1/uXpt1 ==
  In1 : Inport  Port=1  LatchInput=off
  Integrator : Integrator  ExternalReset=none  InitialConditionSource=internal  InitialCondition=vE(1)  LimitOutput=off  UpperSaturationLimit=inf  LowerSaturationLimit=-inf  ShowSaturationPort=off  ShowStatePort=off  AbsoluteTolerance=auto
  Sum : Sum  Inputs=|+-  SaturateOnIntegerOverflow=on
  pt1Const : Gain  Gain=1  Multiplication=Element-wise(K.*u)  SaturateOnIntegerOverflow=on
  pt1Time : Gain  Gain=1/tauAgLp  Multiplication=Element-wise(K.*u)  SaturateOnIntegerOverflow=on
  Out1 : Outport  Port=1
  wires:
  In1/1 -> pt1Const/1
  Integrator/1 -> Sum/2, Out1/1
  pt1Const/1 -> Sum/1
  Sum/1 -> pt1Time/1
  pt1Time/1 -> Integrator/1

== system RotaryWingSim/RBM/6DoF (Euler Angles)1/uYpt1 ==
  In1 : Inport  Port=1  LatchInput=off
  Integrator : Integrator  ExternalReset=none  InitialConditionSource=internal  InitialCondition=vE(2)  LimitOutput=off  UpperSaturationLimit=inf  LowerSaturationLimit=-inf  ShowSaturationPort=off  ShowStatePort=off  AbsoluteTolerance=auto
  Sum : Sum  Inputs=|+-  SaturateOnIntegerOverflow=on
  pt1Const : Gain  Gain=1  Multiplication=Element-wise(K.*u)  SaturateOnIntegerOverflow=on
  pt1Time : Gain  Gain=1/tauAgLp  Multiplication=Element-wise(K.*u)  SaturateOnIntegerOverflow=on
  Out1 : Outport  Port=1
  wires:
  In1/1 -> pt1Const/1
  Integrator/1 -> Sum/2, Out1/1
  pt1Const/1 -> Sum/1
  Sum/1 -> pt1Time/1
  pt1Time/1 -> Integrator/1

== system RotaryWingSim/RBM/6DoF (Euler Angles)1/uZpt1 ==
  In1 : Inport  Port=1  LatchInput=off
  Integrator : Integrator  ExternalReset=none  InitialConditionSource=internal  InitialCondition=vE(3)  LimitOutput=off  UpperSaturationLimit=inf  LowerSaturationLimit=-inf  ShowSaturationPort=off  ShowStatePort=off  AbsoluteTolerance=auto
  Sum : Sum  Inputs=|+-  SaturateOnIntegerOverflow=on
  pt1Const : Gain  Gain=-1  Multiplication=Element-wise(K.*u)  SaturateOnIntegerOverflow=on
  pt1Time : Gain  Gain=1/tauAgLp  Multiplication=Element-wise(K.*u)  SaturateOnIntegerOverflow=on
  Out1 : Outport  Port=1
  wires:
  In1/1 -> pt1Const/1
  Integrator/1 -> Sum/2, Out1/1
  pt1Const/1 -> Sum/1
  Sum/1 -> pt1Time/1
  pt1Time/1 -> Integrator/1
